simulink model "buck_ss_3_digital"  (R2020a)
settings: Solver=VariableStepAuto  StartTime=0.0  StopTime=0.1  RelTol=1e-3
undefined symbols (not defined in the file): DiscIntNeverNeededParam
libraries: powerlib x9, simulink_extras x1, powerlib_meascontrol x1
settings Model: Creator=ayanc  LastModifiedBy=ayanc
settings SolverCC: ZeroCrossAlgorithm=Adaptive
settings DebuggingCC: IgnoredZcDiagnostic=none

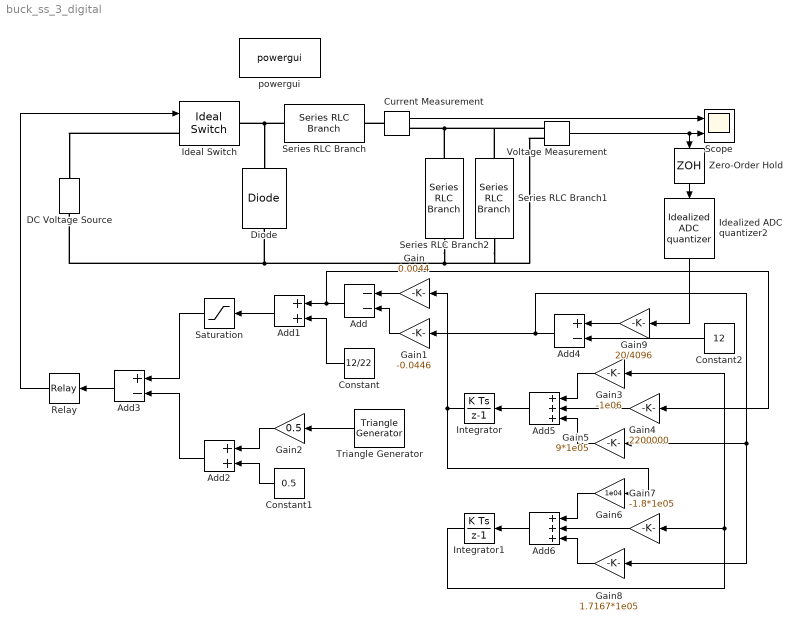
== system buck_ss_3_digital ==
  Add : Sum  Inputs=--
  Add1 : Sum
  Add2 : Sum
  Add3 : Sum  Inputs=+-
  Add4 : Sum  Inputs=+-
  Add5 : Sum  Inputs=+++
  Add6 : Sum  Inputs=+++
  Constant : Constant  Value=12/22
  Constant1 : Constant  Value=0.5
  Constant2 : Constant  Value=12
  Current Measurement : powerlib/Measurements/Current Measurement  PhasorSimulation=off  OutputType=Complex  PSBequivalent=0
  DC Voltage Source : powerlib/Electrical Sources/DC Voltage Source  Amplitude=22  Measurements=None
  Diode : powerlib/Power Electronics/Diode  Ron=0  Lon=0  Vf=0  IC=0  UseSnubber=0  Rs=inf  Cs=0  Measurements=off
  Gain : Gain  Gain=0.0044
  Gain1 : Gain  Gain=-0.0446
  Gain2 : Gain  Gain=0.5
  Gain3 : Gain  Gain=-1e06
  Gain4 : Gain  Gain=2200000
  Gain5 : Gain  Gain=9*1e05
  Gain6 : Gain  Gain=1e04
  Gain7 : Gain  Gain=-1.8*1e05
  Gain8 : Gain  Gain=1.7167*1e05
  Gain9 : Gain  Gain=20/4096
  Ideal Switch : powerlib/Power Electronics/Ideal Switch  Ron=0  Lon=0  IC=0  Rs=inf  Cs=inf  Measurements=off
  Idealized ADC quantizer2 : simulink_extras/Additional Discrete/Idealized ADC quantizer  NumberOfConverterBits=12  Vmin=0  Vmax=20  OutputDataType=int16  OutputNegativeValues=off
  Integrator : DiscreteIntegrator  SampleTime=1e-8  ICPrevOutput=DiscIntNeverNeededParam  ICPrevScaledInput=DiscIntNeverNeededParam  mask(DiscretizedDiscreteIntegrator){}
      mask init:
      | %zoh
  Integrator1 : DiscreteIntegrator  SampleTime=1e-8  ICPrevOutput=DiscIntNeverNeededParam  ICPrevScaledInput=DiscIntNeverNeededParam  mask(DiscretizedDiscreteIntegrator){}
      mask init:
      | %zoh
  Relay : Relay
  Saturation : Saturate  UpperLimit=1  LowerLimit=0  ZeroCross=off
  Scope : Scope  NumInputPorts=2
  Series RLC Branch : powerlib/Elements/Series RLC Branch  LConnTagsString=__new0  RConnTagsString=__new0  BranchType=L  Resistance=1  Inductance=10e-06  SetiL0=off  InitialCurrent=0  Capacitance=1e-6  Setx0=off  InitialVoltage=0  Measurements=None
  Series RLC Branch1 : powerlib/Elements/Series RLC Branch  LConnTagsString=__new0  RConnTagsString=__new0  BranchType=R  Resistance=1.2  Inductance=1e-3  SetiL0=off  InitialCurrent=0  Capacitance=1e-6  Setx0=off  InitialVoltage=0  Measurements=None
  Series RLC Branch2 : powerlib/Elements/Series RLC Branch  LConnTagsString=__new0  RConnTagsString=__new0  BranchType=C  Resistance=1  Inductance=1e-3  SetiL0=off  InitialCurrent=0  Capacitance=100e-06  Setx0=off  InitialVoltage=0  Measurements=None
  Triangle Generator : powerlib_meascontrol/Pulse & Signal Generators/Triangle Generator  Freq=500e3  Phase=90  Ts=0
  Voltage Measurement : powerlib/Measurements/Voltage Measurement  PhasorSimulation=off  OutputType=Complex  PSBequivalent=0
  Zero-Order Hold : ZeroOrderHold  SampleTime=1e-8
  powergui : powerlib/powergui  Priority=1  SimulationMode=Continuous  SampleTime=50e-6  frequency=60  Iterations=50  frequencyindice=0  Pbase=100e6  ErrMax=1e-4  UnitsV=kV  UnitsW=MW  buscounter=0  FunctionMessages=off  echomessages=off  EnableUseOfTLC=off  CurrentSourceSwitches=off  DisableSnubberDevices=off  DisableRonSwitches=off  DisableVfSwitches=off  DisplayEquations=off  AutomaticDiscreteSolvers=off  SolverType=Tustin/Backward Euler (TBE)  Interpol=off  ExternalGateDelay=off  methode=off  Ts=100  x0status=blocks  SPID=on  SwTol=0  HookPort=off  NonlinearTolerance=1e-4  nMaxIteration=100  ContinueOnMaxIteration=off  RestoreLinks=warning  ResistiveCurrentMeasurement=off  Frange=[0:2:500]  Ylog=off  Xlog=on  ShowGrid=off  save=off  variable=ZData  structure=0  ZoomFFT=off  StartTime=0.0  cycles=1  DisplayStyle=1  fundamental=60  FreqAxis=off  MaxFrequency=1000  frequencyindicesteady=1  RmsSteady=1  display=off
  wires:
  Relay/1 -> Ideal Switch/1
  Constant/1 -> Add1/2
  Triangle Generator/1 -> Gain2/1
  Saturation/1 -> Add3/1
  Voltage Measurement/1 -> Zero-Order Hold/1, Scope/2
  Add3/1 -> Relay/1
  Constant1/1 -> Add2/2
  Add/1 -> Gain4/1, Add1/1
  Add1/1 -> Saturation/1
  Add2/1 -> Add3/2
  Current Measurement/1 -> Scope/1
  Gain2/1 -> Add2/1
  Gain/1 -> Add/1
  Gain1/1 -> Add/2
  Add4/1 -> Gain8/1, Gain5/1, Gain1/1
  Constant2/1 -> Add4/2
  Integrator/1 -> Gain6/1, Gain/1
  Add5/1 -> Integrator/1
  Add6/1 -> Integrator1/1
  Gain3/1 -> Add5/1
  Integrator1/1 -> Gain7/1, Gain3/1
  Gain4/1 -> Add5/2
  Gain5/1 -> Add5/3
  Gain8/1 -> Add6/3
  Gain6/1 -> Add6/1
  Gain7/1 -> Add6/2
  Zero-Order Hold/1 -> Idealized ADC quantizer2/1
  Gain9/1 -> Add4/1
  Idealized ADC quantizer2/1 -> Gain9/1
  connections:
  Series RLC Branch2/RConn1 -- Diode/LConn1 -- DC Voltage Source/LConn1 -- Voltage Measurement/LConn2 -- Series RLC Branch1/RConn1
  Series RLC Branch2/LConn1 -- Current Measurement/RConn1 -- Voltage Measurement/LConn1 -- Series RLC Branch1/LConn1
  Series RLC Branch/LConn1 -- Ideal Switch/RConn1 -- Diode/RConn1
  Ideal Switch/LConn1 -- DC Voltage Source/RConn1
  Current Measurement/LConn1 -- Series RLC Branch/RConn1
